simulink model "Linear_HydroDyn"  (R2022a)
settings: Solver=VariableStepAuto  StartTime=0.16733  StopTime=3000.0185  RelTol=1e-3
undefined symbols (not defined in the file): A_HD, B_HD, C_HD, HD_FOP
settings Model: Creator=ianam  LastModifiedBy=ianam
settings DataIOCC: InitialState=IC  LoadInitialState=on
settings DebuggingCC: UnderSpecifiedDataTypeMsg=error  UnderSpecifiedDimensionMsg=error

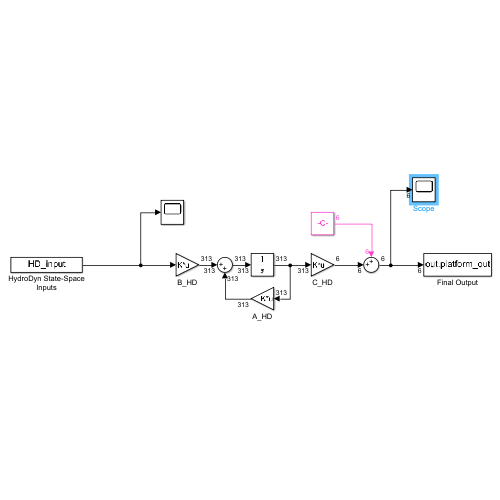
[thumbnail: Simulink's stored preview of the top-level diagram]
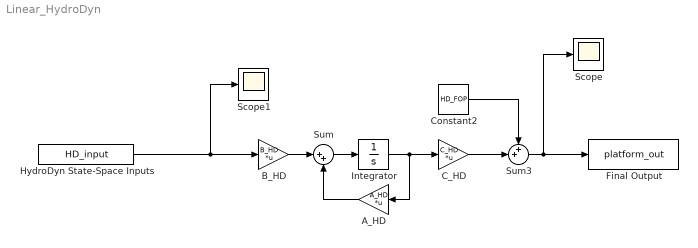
== system Linear_HydroDyn ==
  A_HD : Gain  Gain=A_HD  Multiplication=Matrix(K*u)
  B_HD : Gain  Gain=B_HD  Multiplication=Matrix(K*u)
  C_HD : Gain  Gain=C_HD  Multiplication=Matrix(K*u)
  Constant2 : Constant  Value=HD_FOP
  Final Output : ToWorkspace  VariableName=platform_out  SaveFormat=Timeseries  SampleTime=-1
  HydroDyn State-Space Inputs : FromWorkspace  VariableName=HD_input
  Integrator : Integrator
  Scope : Scope
  Scope1 : Scope
  Sum : Sum  Inputs=|++
  Sum3 : Sum  Inputs=++|
  wires:
  Sum/1 -> Integrator/1
  Integrator/1 -> C_HD/1, A_HD/1
  A_HD/1 -> Sum/2
  B_HD/1 -> Sum/1
  HydroDyn State-Space Inputs/1 -> Scope1/1, B_HD/1
  C_HD/1 -> Sum3/2
  Sum3/1 -> Final Output/1, Scope/1
  Constant2/1 -> Sum3/1
